simulink model "heart_model"  (Simulink 8.5)
settings: Solver=ode3  StartTime=0.0  StopTime=size(sasignal,1)  FixedStep=1  RelTol=1e-6  AbsTol=1e-6
undefined symbols (not defined in the file or in its folder): beta1, beta3, beta4, delay, gain
libraries: simulink x40, dspsrcs4 x1
(part 2 of 5)

== system heart_model/Heart Model/VENTRICLE/LV (20) ==
  stim : Inport
  I_st : Inport  Port=2
  vin : Inport  Port=3
  win : Inport  Port=4
  Data Type Conversion : DataTypeConversion  OutMin=[0]  OutMax=[1]  OutDataTypeStr=double  LockScale=on
  Data Type Conversion1 : DataTypeConversion  OutMin=[0]  OutMax=[1]  OutDataTypeStr=double  LockScale=on
  Data Type Conversion2 : DataTypeConversion  OutMin=[0]  OutMax=[1]  OutDataTypeStr=double  LockScale=on
  Event generator : Stateflow chart  TreatAsAtomicUnit=on
  Hybrid set : Stateflow chart  TreatAsAtomicUnit=on
  Mux : Mux  Inputs=5
  Subsystem3 : Subsystem
  vout : Outport
  wires:
  Data Type Conversion2/1 -> Mux/3
  Data Type Conversion1/1 -> Mux/2
  Event generator/3(event3) -> Data Type Conversion2/1
  Event generator/2(event2) -> Data Type Conversion1/1
  Data Type Conversion/1 -> Mux/1
  Event generator/1(event1) -> Data Type Conversion/1
  stim/1 -> Mux/5, Mux/4
  Mux/1 -> Hybrid set/Trigger
  win/1 -> Subsystem3/7(win)
  vin/1 -> Subsystem3/6(vin)
  Hybrid set/3(vno) -> Subsystem3/5(vno)
  I_st/1 -> Subsystem3/4(I_st)
  Subsystem3/1(v) -> vout/1
  Hybrid set/1(q) -> Subsystem3/1(q)
  Subsystem3/2(vnext) -> Event generator/1(v), Hybrid set/1(v)
  Hybrid set/2(vreset) -> Subsystem3/2(vreset)
  Hybrid set/4(reset) -> Subsystem3/3(reset)

== system heart_model/Heart Model/VENTRICLE/LVA (16) ==
  stim : Inport
  I_st : Inport  Port=2
  vin : Inport  Port=3
  win : Inport  Port=4
  Data Type Conversion : DataTypeConversion  OutMin=[0]  OutMax=[1]  OutDataTypeStr=double  LockScale=on
  Data Type Conversion1 : DataTypeConversion  OutMin=[0]  OutMax=[1]  OutDataTypeStr=double  LockScale=on
  Data Type Conversion2 : DataTypeConversion  OutMin=[0]  OutMax=[1]  OutDataTypeStr=double  LockScale=on
  Event generator : Stateflow chart  TreatAsAtomicUnit=on
  Hybrid set : Stateflow chart  TreatAsAtomicUnit=on
  Mux : Mux  Inputs=5
  Subsystem3 : Subsystem
  vout : Outport
  wires:
  Data Type Conversion2/1 -> Mux/3
  Data Type Conversion1/1 -> Mux/2
  Event generator/3(event3) -> Data Type Conversion2/1
  Event generator/2(event2) -> Data Type Conversion1/1
  Data Type Conversion/1 -> Mux/1
  Event generator/1(event1) -> Data Type Conversion/1
  stim/1 -> Mux/5, Mux/4
  Mux/1 -> Hybrid set/Trigger
  win/1 -> Subsystem3/7(win)
  vin/1 -> Subsystem3/6(vin)
  Hybrid set/3(vno) -> Subsystem3/5(vno)
  I_st/1 -> Subsystem3/4(I_st)
  Subsystem3/1(v) -> vout/1
  Hybrid set/1(q) -> Subsystem3/1(q)
  Subsystem3/2(vnext) -> Event generator/1(v), Hybrid set/1(v)
  Hybrid set/2(vreset) -> Subsystem3/2(vreset)
  Hybrid set/4(reset) -> Subsystem3/3(reset)

== system heart_model/Heart Model/VENTRICLE/LV_m (19) ==
  stim : Inport
  I_st : Inport  Port=2
  vin : Inport  Port=3
  win : Inport  Port=4
  Data Type Conversion : DataTypeConversion  OutMin=[0]  OutMax=[1]  OutDataTypeStr=double  LockScale=on
  Data Type Conversion1 : DataTypeConversion  OutMin=[0]  OutMax=[1]  OutDataTypeStr=double  LockScale=on
  Data Type Conversion2 : DataTypeConversion  OutMin=[0]  OutMax=[1]  OutDataTypeStr=double  LockScale=on
  Event generator : Stateflow chart  TreatAsAtomicUnit=on
  Hybrid set : Stateflow chart  TreatAsAtomicUnit=on
  Mux : Mux  Inputs=5
  Subsystem3 : Subsystem
  vout : Outport
  wires:
  Data Type Conversion2/1 -> Mux/3
  Data Type Conversion1/1 -> Mux/2
  Event generator/3(event3) -> Data Type Conversion2/1
  Event generator/2(event2) -> Data Type Conversion1/1
  Data Type Conversion/1 -> Mux/1
  Event generator/1(event1) -> Data Type Conversion/1
  stim/1 -> Mux/5, Mux/4
  Mux/1 -> Hybrid set/Trigger
  win/1 -> Subsystem3/7(win)
  vin/1 -> Subsystem3/6(vin)
  Hybrid set/3(vno) -> Subsystem3/5(vno)
  I_st/1 -> Subsystem3/4(I_st)
  Subsystem3/1(v) -> vout/1
  Hybrid set/1(q) -> Subsystem3/1(q)
  Subsystem3/2(vnext) -> Event generator/1(v), Hybrid set/1(v)
  Hybrid set/2(vreset) -> Subsystem3/2(vreset)
  Hybrid set/4(reset) -> Subsystem3/3(reset)

== system heart_model/Heart Model/VENTRICLE/RBB (12) ==
  stim : Inport
  I_st : Inport  Port=2
  vin : Inport  Port=3
  win : Inport  Port=4
  Data Type Conversion : DataTypeConversion  OutMin=[0]  OutMax=[1]  OutDataTypeStr=double  LockScale=on
  Data Type Conversion1 : DataTypeConversion  OutMin=[0]  OutMax=[1]  OutDataTypeStr=double  LockScale=on
  Data Type Conversion2 : DataTypeConversion  OutMin=[0]  OutMax=[1]  OutDataTypeStr=double  LockScale=on
  Event generator : Stateflow chart  TreatAsAtomicUnit=on
  Hybrid set : Stateflow chart  TreatAsAtomicUnit=on
  Mux : Mux  Inputs=5
  Subsystem3 : Subsystem
  vout : Outport
  wires:
  Data Type Conversion2/1 -> Mux/3
  Data Type Conversion1/1 -> Mux/2
  Event generator/3(event3) -> Data Type Conversion2/1
  Event generator/2(event2) -> Data Type Conversion1/1
  Data Type Conversion/1 -> Mux/1
  Event generator/1(event1) -> Data Type Conversion/1
  stim/1 -> Mux/5, Mux/4
  Mux/1 -> Hybrid set/Trigger
  win/1 -> Subsystem3/7(win)
  vin/1 -> Subsystem3/6(vin)
  Hybrid set/3(vno) -> Subsystem3/5(vno)
  I_st/1 -> Subsystem3/4(I_st)
  Subsystem3/1(v) -> vout/1
  Hybrid set/1(q) -> Subsystem3/1(q)
  Subsystem3/2(vnext) -> Event generator/1(v), Hybrid set/1(v)
  Hybrid set/2(vreset) -> Subsystem3/2(vreset)
  Hybrid set/4(reset) -> Subsystem3/3(reset)

== system heart_model/Heart Model/VENTRICLE/RBB_m (11) ==
  stim : Inport
  I_st : Inport  Port=2
  vin : Inport  Port=3
  win : Inport  Port=4
  Data Type Conversion : DataTypeConversion  OutMin=[0]  OutMax=[1]  OutDataTypeStr=double  LockScale=on
  Data Type Conversion1 : DataTypeConversion  OutMin=[0]  OutMax=[1]  OutDataTypeStr=double  LockScale=on
  Data Type Conversion2 : DataTypeConversion  OutMin=[0]  OutMax=[1]  OutDataTypeStr=double  LockScale=on
  Event generator : Stateflow chart  TreatAsAtomicUnit=on
  Hybrid set : Stateflow chart  TreatAsAtomicUnit=on
  Mux : Mux  Inputs=5
  Subsystem3 : Subsystem
  vout : Outport
  wires:
  Data Type Conversion2/1 -> Mux/3
  Data Type Conversion1/1 -> Mux/2
  Event generator/3(event3) -> Data Type Conversion2/1
  Event generator/2(event2) -> Data Type Conversion1/1
  Data Type Conversion/1 -> Mux/1
  Event generator/1(event1) -> Data Type Conversion/1
  stim/1 -> Mux/5, Mux/4
  Mux/1 -> Hybrid set/Trigger
  win/1 -> Subsystem3/7(win)
  vin/1 -> Subsystem3/6(vin)
  Hybrid set/3(vno) -> Subsystem3/5(vno)
  I_st/1 -> Subsystem3/4(I_st)
  Subsystem3/1(v) -> vout/1
  Hybrid set/1(q) -> Subsystem3/1(q)
  Subsystem3/2(vnext) -> Event generator/1(v), Hybrid set/1(v)
  Hybrid set/2(vreset) -> Subsystem3/2(vreset)
  Hybrid set/4(reset) -> Subsystem3/3(reset)

== system heart_model/Heart Model/VENTRICLE/RV (18) ==
  stim : Inport
  I_st : Inport  Port=2
  vin : Inport  Port=3
  win : Inport  Port=4
  Data Type Conversion : DataTypeConversion  OutMin=[0]  OutMax=[1]  OutDataTypeStr=double  LockScale=on
  Data Type Conversion1 : DataTypeConversion  OutMin=[0]  OutMax=[1]  OutDataTypeStr=double  LockScale=on
  Data Type Conversion2 : DataTypeConversion  OutMin=[0]  OutMax=[1]  OutDataTypeStr=double  LockScale=on
  Event generator : Stateflow chart  TreatAsAtomicUnit=on
  Hybrid set : Stateflow chart  TreatAsAtomicUnit=on
  Mux : Mux  Inputs=5
  Subsystem3 : Subsystem
  vout : Outport
  wires:
  Data Type Conversion2/1 -> Mux/3
  Data Type Conversion1/1 -> Mux/2
  Event generator/3(event3) -> Data Type Conversion2/1
  Event generator/2(event2) -> Data Type Conversion1/1
  Data Type Conversion/1 -> Mux/1
  Event generator/1(event1) -> Data Type Conversion/1
  stim/1 -> Mux/5, Mux/4
  Mux/1 -> Hybrid set/Trigger
  win/1 -> Subsystem3/7(win)
  vin/1 -> Subsystem3/6(vin)
  Hybrid set/3(vno) -> Subsystem3/5(vno)
  I_st/1 -> Subsystem3/4(I_st)
  Subsystem3/1(v) -> vout/1
  Hybrid set/1(q) -> Subsystem3/1(q)
  Subsystem3/2(vnext) -> Event generator/1(v), Hybrid set/1(v)
  Hybrid set/2(vreset) -> Subsystem3/2(vreset)
  Hybrid set/4(reset) -> Subsystem3/3(reset)

== system heart_model/Heart Model/VENTRICLE/RVA (15) ==
  stim : Inport
  I_st : Inport  Port=2
  vin : Inport  Port=3
  win : Inport  Port=4
  Data Type Conversion : DataTypeConversion  OutMin=[0]  OutMax=[1]  OutDataTypeStr=double  LockScale=on
  Data Type Conversion1 : DataTypeConversion  OutMin=[0]  OutMax=[1]  OutDataTypeStr=double  LockScale=on
  Data Type Conversion2 : DataTypeConversion  OutMin=[0]  OutMax=[1]  OutDataTypeStr=double  LockScale=on
  Event generator : Stateflow chart  TreatAsAtomicUnit=on
  Hybrid set : Stateflow chart  TreatAsAtomicUnit=on
  Mux : Mux  Inputs=5
  Subsystem3 : Subsystem
  vout : Outport
  wires:
  Data Type Conversion2/1 -> Mux/3
  Data Type Conversion1/1 -> Mux/2
  Event generator/3(event3) -> Data Type Conversion2/1
  Event generator/2(event2) -> Data Type Conversion1/1
  Data Type Conversion/1 -> Mux/1
  Event generator/1(event1) -> Data Type Conversion/1
  stim/1 -> Mux/5, Mux/4
  Mux/1 -> Hybrid set/Trigger
  win/1 -> Subsystem3/7(win)
  vin/1 -> Subsystem3/6(vin)
  Hybrid set/3(vno) -> Subsystem3/5(vno)
  I_st/1 -> Subsystem3/4(I_st)
  Subsystem3/1(v) -> vout/1
  Hybrid set/1(q) -> Subsystem3/1(q)
  Subsystem3/2(vnext) -> Event generator/1(v), Hybrid set/1(v)
  Hybrid set/2(vreset) -> Subsystem3/2(vreset)
  Hybrid set/4(reset) -> Subsystem3/3(reset)

== system heart_model/Heart Model/VENTRICLE/RV_m (17) ==
  stim : Inport
  I_st : Inport  Port=2
  vin : Inport  Port=3
  win : Inport  Port=4
  Data Type Conversion : DataTypeConversion  OutMin=[0]  OutMax=[1]  OutDataTypeStr=double  LockScale=on
  Data Type Conversion1 : DataTypeConversion  OutMin=[0]  OutMax=[1]  OutDataTypeStr=double  LockScale=on
  Data Type Conversion2 : DataTypeConversion  OutMin=[0]  OutMax=[1]  OutDataTypeStr=double  LockScale=on
  Event generator : Stateflow chart  TreatAsAtomicUnit=on
  Hybrid set : Stateflow chart  TreatAsAtomicUnit=on
  Mux : Mux  Inputs=5
  Subsystem3 : Subsystem
  vout : Outport
  wires:
  Data Type Conversion2/1 -> Mux/3
  Data Type Conversion1/1 -> Mux/2
  Event generator/3(event3) -> Data Type Conversion2/1
  Event generator/2(event2) -> Data Type Conversion1/1
  Data Type Conversion/1 -> Mux/1
  Event generator/1(event1) -> Data Type Conversion/1
  stim/1 -> Mux/5, Mux/4
  Mux/1 -> Hybrid set/Trigger
  win/1 -> Subsystem3/7(win)
  vin/1 -> Subsystem3/6(vin)
  Hybrid set/3(vno) -> Subsystem3/5(vno)
  I_st/1 -> Subsystem3/4(I_st)
  Subsystem3/1(v) -> vout/1
  Hybrid set/1(q) -> Subsystem3/1(q)
  Subsystem3/2(vnext) -> Event generator/1(v), Hybrid set/1(v)
  Hybrid set/2(vreset) -> Subsystem3/2(vreset)
  Hybrid set/4(reset) -> Subsystem3/3(reset)

== system heart_model/Heart Model/VENTRICLE/SEP_LV (27) ==
  stim : Inport
  I_st : Inport  Port=2
  vin : Inport  Port=3
  win : Inport  Port=4
  Data Type Conversion : DataTypeConversion  OutMin=[0]  OutMax=[1]  OutDataTypeStr=double  LockScale=on
  Data Type Conversion1 : DataTypeConversion  OutMin=[0]  OutMax=[1]  OutDataTypeStr=double  LockScale=on
  Data Type Conversion2 : DataTypeConversion  OutMin=[0]  OutMax=[1]  OutDataTypeStr=double  LockScale=on
  Event generator : Stateflow chart  TreatAsAtomicUnit=on
  Hybrid set : Stateflow chart  TreatAsAtomicUnit=on
  Mux : Mux  Inputs=5
  Subsystem3 : Subsystem
  vout : Outport
  wires:
  Data Type Conversion2/1 -> Mux/3
  Data Type Conversion1/1 -> Mux/2
  Event generator/3(event3) -> Data Type Conversion2/1
  Event generator/2(event2) -> Data Type Conversion1/1
  Data Type Conversion/1 -> Mux/1
  Event generator/1(event1) -> Data Type Conversion/1
  stim/1 -> Mux/5, Mux/4
  Mux/1 -> Hybrid set/Trigger
  win/1 -> Subsystem3/7(win)
  vin/1 -> Subsystem3/6(vin)
  Hybrid set/3(vno) -> Subsystem3/5(vno)
  I_st/1 -> Subsystem3/4(I_st)
  Subsystem3/1(v) -> vout/1
  Hybrid set/1(q) -> Subsystem3/1(q)
  Subsystem3/2(vnext) -> Event generator/1(v), Hybrid set/1(v)
  Hybrid set/2(vreset) -> Subsystem3/2(vreset)
  Hybrid set/4(reset) -> Subsystem3/3(reset)

== system heart_model/Heart Model/VENTRICLE/SEP_LV_m (26) ==
  stim : Inport
  I_st : Inport  Port=2
  vin : Inport  Port=3
  win : Inport  Port=4
  Data Type Conversion : DataTypeConversion  OutMin=[0]  OutMax=[1]  OutDataTypeStr=double  LockScale=on
  Data Type Conversion1 : DataTypeConversion  OutMin=[0]  OutMax=[1]  OutDataTypeStr=double  LockScale=on
  Data Type Conversion2 : DataTypeConversion  OutMin=[0]  OutMax=[1]  OutDataTypeStr=double  LockScale=on
  Event generator : Stateflow chart  TreatAsAtomicUnit=on
  Hybrid set : Stateflow chart  TreatAsAtomicUnit=on
  Mux : Mux  Inputs=5
  Subsystem3 : Subsystem
  vout : Outport
  wires:
  Data Type Conversion2/1 -> Mux/3
  Data Type Conversion1/1 -> Mux/2
  Event generator/3(event3) -> Data Type Conversion2/1
  Event generator/2(event2) -> Data Type Conversion1/1
  Data Type Conversion/1 -> Mux/1
  Event generator/1(event1) -> Data Type Conversion/1
  stim/1 -> Mux/5, Mux/4
  Mux/1 -> Hybrid set/Trigger
  win/1 -> Subsystem3/7(win)
  vin/1 -> Subsystem3/6(vin)
  Hybrid set/3(vno) -> Subsystem3/5(vno)
  I_st/1 -> Subsystem3/4(I_st)
  Subsystem3/1(v) -> vout/1
  Hybrid set/1(q) -> Subsystem3/1(q)
  Subsystem3/2(vnext) -> Event generator/1(v), Hybrid set/1(v)
  Hybrid set/2(vreset) -> Subsystem3/2(vreset)
  Hybrid set/4(reset) -> Subsystem3/3(reset)

== system heart_model/Heart Model/VENTRICLE/SEP_RV (25) ==
  stim : Inport
  I_st : Inport  Port=2
  vin : Inport  Port=3
  win : Inport  Port=4
  Data Type Conversion : DataTypeConversion  OutMin=[0]  OutMax=[1]  OutDataTypeStr=double  LockScale=on
  Data Type Conversion1 : DataTypeConversion  OutMin=[0]  OutMax=[1]  OutDataTypeStr=double  LockScale=on
  Data Type Conversion2 : DataTypeConversion  OutMin=[0]  OutMax=[1]  OutDataTypeStr=double  LockScale=on
  Event generator : Stateflow chart  TreatAsAtomicUnit=on
  Hybrid set : Stateflow chart  TreatAsAtomicUnit=on
  Mux : Mux  Inputs=5
  Subsystem3 : Subsystem
  vout : Outport
  wires:
  Data Type Conversion2/1 -> Mux/3
  Data Type Conversion1/1 -> Mux/2
  Event generator/3(event3) -> Data Type Conversion2/1
  Event generator/2(event2) -> Data Type Conversion1/1
  Data Type Conversion/1 -> Mux/1
  Event generator/1(event1) -> Data Type Conversion/1
  stim/1 -> Mux/5, Mux/4
  Mux/1 -> Hybrid set/Trigger
  win/1 -> Subsystem3/7(win)
  vin/1 -> Subsystem3/6(vin)
  Hybrid set/3(vno) -> Subsystem3/5(vno)
  I_st/1 -> Subsystem3/4(I_st)
  Subsystem3/1(v) -> vout/1
  Hybrid set/1(q) -> Subsystem3/1(q)
  Subsystem3/2(vnext) -> Event generator/1(v), Hybrid set/1(v)
  Hybrid set/2(vreset) -> Subsystem3/2(vreset)
  Hybrid set/4(reset) -> Subsystem3/3(reset)

== system heart_model/Heart Model/VENTRICLE/SEP_RV_m (24) ==
  stim : Inport
  I_st : Inport  Port=2
  vin : Inport  Port=3
  win : Inport  Port=4
  Data Type Conversion : DataTypeConversion  OutMin=[0]  OutMax=[1]  OutDataTypeStr=double  LockScale=on
  Data Type Conversion1 : DataTypeConversion  OutMin=[0]  OutMax=[1]  OutDataTypeStr=double  LockScale=on
  Data Type Conversion2 : DataTypeConversion  OutMin=[0]  OutMax=[1]  OutDataTypeStr=double  LockScale=on
  Event generator : Stateflow chart  TreatAsAtomicUnit=on
  Hybrid set : Stateflow chart  TreatAsAtomicUnit=on
  Mux : Mux  Inputs=5
  Subsystem3 : Subsystem
  vout : Outport
  wires:
  Data Type Conversion2/1 -> Mux/3
  Data Type Conversion1/1 -> Mux/2
  Event generator/3(event3) -> Data Type Conversion2/1
  Event generator/2(event2) -> Data Type Conversion1/1
  Data Type Conversion/1 -> Mux/1
  Event generator/1(event1) -> Data Type Conversion/1
  stim/1 -> Mux/5, Mux/4
  Mux/1 -> Hybrid set/Trigger
  win/1 -> Subsystem3/7(win)
  vin/1 -> Subsystem3/6(vin)
  Hybrid set/3(vno) -> Subsystem3/5(vno)
  I_st/1 -> Subsystem3/4(I_st)
  Subsystem3/1(v) -> vout/1
  Hybrid set/1(q) -> Subsystem3/1(q)
  Subsystem3/2(vnext) -> Event generator/1(v), Hybrid set/1(v)
  Hybrid set/2(vreset) -> Subsystem3/2(vreset)
  Hybrid set/4(reset) -> Subsystem3/3(reset)

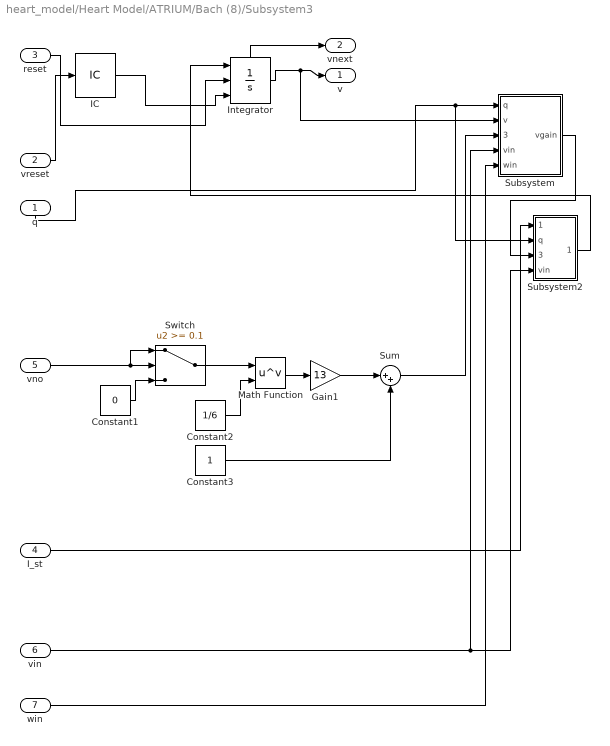
== system heart_model/Heart Model/ATRIUM/Bach (8)/Subsystem3 ==
  q : Inport
  vreset : Inport  Port=2
  reset : Inport  Port=3
  I_st : Inport  Port=4
  vno : Inport  Port=5
  vin : Inport  Port=6
  win : Inport  Port=7
  Constant1 : Constant  Value=0
  Constant2 : Constant  Value=1/6
  Constant3 : Constant
  Gain1 : Gain  Gain=13
  IC : InitialCondition  Value=0
  Integrator : Integrator  ExternalReset=either  InitialConditionSource=external  LimitOutput=on  UpperSaturationLimit=138  ShowStatePort=on
  Math Function : Math  Operator=pow  SaturateOnIntegerOverflow=on
  Subsystem : Subsystem
  Subsystem2 : Subsystem
  Sum : Sum  Inputs=|++
  Switch : Switch  Threshold=0.1
  v : Outport
  vnext : Outport  Port=2
  wires:
  win/1 -> Subsystem/5(win)
  vin/1 -> Subsystem/4(vin), Subsystem2/4(vin)
  Integrator/State -> vnext/1
  Constant1/1 -> Switch/3
  vno/1 -> Switch/1, Switch/2
  Sum/1 -> Subsystem/3(f(vno))
  Switch/1 -> Math Function/1
  Constant3/1 -> Sum/2
  Gain1/1 -> Sum/1
  Math Function/1 -> Gain1/1
  Constant2/1 -> Math Function/2
  I_st/1 -> Subsystem2/1(I_st)
  reset/1 -> Integrator/2
  vreset/1 -> IC/1
  Subsystem2/1(vint) -> Integrator/1
  Subsystem/1(vgain) -> Subsystem2/3(vgain)
  Integrator/1 -> Subsystem/2(v), v/1
  IC/1 -> Integrator/3
  q/1 -> Subsystem/1(q), Subsystem2/2(q)

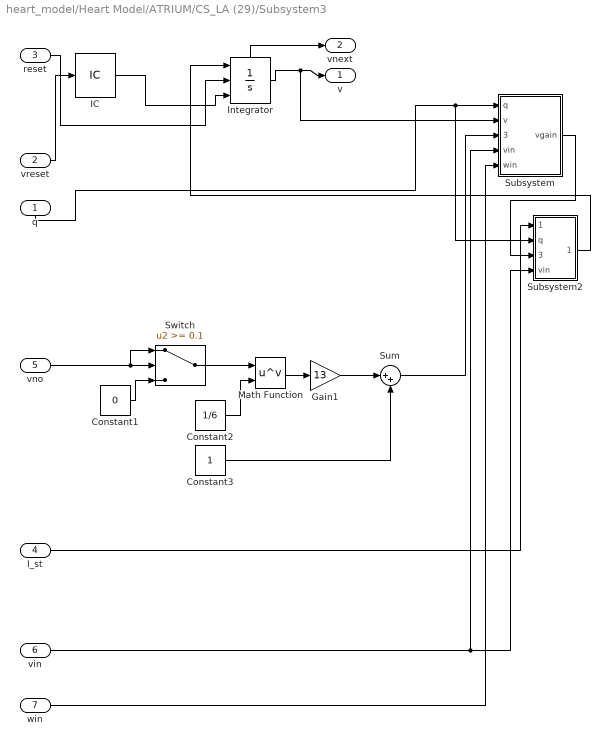
== system heart_model/Heart Model/ATRIUM/CS_LA (29)/Subsystem3 ==
  q : Inport
  vreset : Inport  Port=2
  reset : Inport  Port=3
  I_st : Inport  Port=4
  vno : Inport  Port=5
  vin : Inport  Port=6
  win : Inport  Port=7
  Constant1 : Constant  Value=0
  Constant2 : Constant  Value=1/6
  Constant3 : Constant
  Gain1 : Gain  Gain=13
  IC : InitialCondition  Value=0
  Integrator : Integrator  ExternalReset=either  InitialConditionSource=external  LimitOutput=on  UpperSaturationLimit=138  ShowStatePort=on
  Math Function : Math  Operator=pow  SaturateOnIntegerOverflow=on
  Subsystem : Subsystem
  Subsystem2 : Subsystem
  Sum : Sum  Inputs=|++
  Switch : Switch  Threshold=0.1
  v : Outport
  vnext : Outport  Port=2
  wires:
  win/1 -> Subsystem/5(win)
  vin/1 -> Subsystem/4(vin), Subsystem2/4(vin)
  Integrator/State -> vnext/1
  Constant1/1 -> Switch/3
  vno/1 -> Switch/1, Switch/2
  Sum/1 -> Subsystem/3(f(vno))
  Switch/1 -> Math Function/1
  Constant3/1 -> Sum/2
  Gain1/1 -> Sum/1
  Math Function/1 -> Gain1/1
  Constant2/1 -> Math Function/2
  I_st/1 -> Subsystem2/1(I_st)
  reset/1 -> Integrator/2
  vreset/1 -> IC/1
  Subsystem2/1(vint) -> Integrator/1
  Subsystem/1(vgain) -> Subsystem2/3(vgain)
  Integrator/1 -> Subsystem/2(v), v/1
  IC/1 -> Integrator/3
  q/1 -> Subsystem/1(q), Subsystem2/2(q)

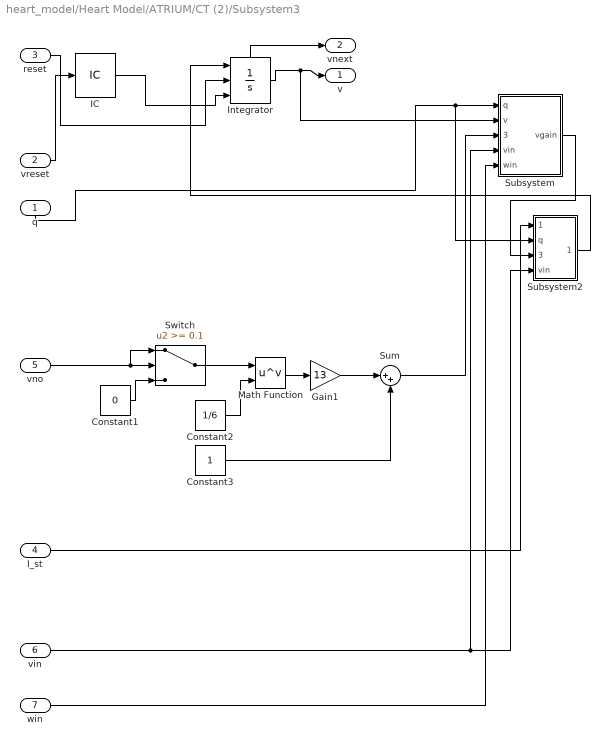
== system heart_model/Heart Model/ATRIUM/CT (2)/Subsystem3 ==
  q : Inport
  vreset : Inport  Port=2
  reset : Inport  Port=3
  I_st : Inport  Port=4
  vno : Inport  Port=5
  vin : Inport  Port=6
  win : Inport  Port=7
  Constant1 : Constant  Value=0
  Constant2 : Constant  Value=1/6
  Constant3 : Constant
  Gain1 : Gain  Gain=13
  IC : InitialCondition  Value=0
  Integrator : Integrator  ExternalReset=either  InitialConditionSource=external  LimitOutput=on  UpperSaturationLimit=138  ShowStatePort=on
  Math Function : Math  Operator=pow  SaturateOnIntegerOverflow=on
  Subsystem : Subsystem
  Subsystem2 : Subsystem
  Sum : Sum  Inputs=|++
  Switch : Switch  Threshold=0.1
  v : Outport
  vnext : Outport  Port=2
  wires:
  win/1 -> Subsystem/5(win)
  vin/1 -> Subsystem/4(vin), Subsystem2/4(vin)
  Integrator/State -> vnext/1
  Constant1/1 -> Switch/3
  vno/1 -> Switch/1, Switch/2
  Sum/1 -> Subsystem/3(f(vno))
  Switch/1 -> Math Function/1
  Constant3/1 -> Sum/2
  Gain1/1 -> Sum/1
  Math Function/1 -> Gain1/1
  Constant2/1 -> Math Function/2
  I_st/1 -> Subsystem2/1(I_st)
  reset/1 -> Integrator/2
  vreset/1 -> IC/1
  Subsystem2/1(vint) -> Integrator/1
  Subsystem/1(vgain) -> Subsystem2/3(vgain)
  Integrator/1 -> Subsystem/2(v), v/1
  IC/1 -> Integrator/3
  q/1 -> Subsystem/1(q), Subsystem2/2(q)

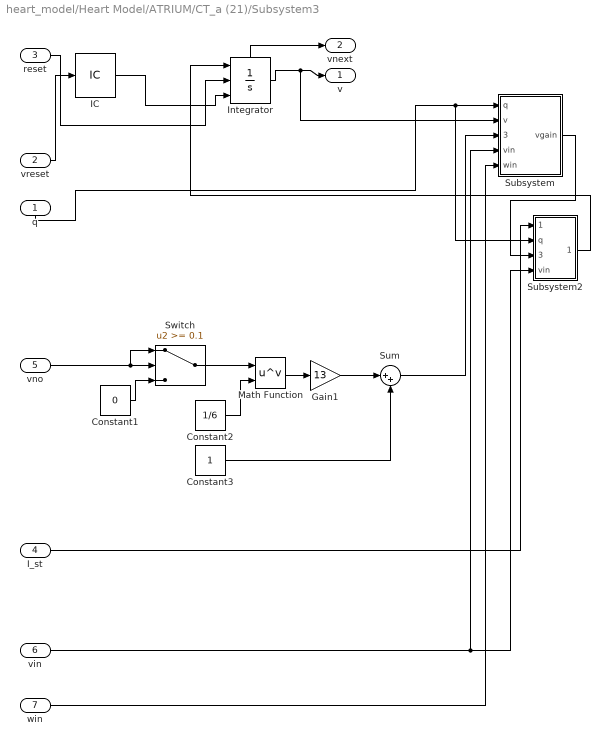
== system heart_model/Heart Model/ATRIUM/CT_a (21)/Subsystem3 ==
  q : Inport
  vreset : Inport  Port=2
  reset : Inport  Port=3
  I_st : Inport  Port=4
  vno : Inport  Port=5
  vin : Inport  Port=6
  win : Inport  Port=7
  Constant1 : Constant  Value=0
  Constant2 : Constant  Value=1/6
  Constant3 : Constant
  Gain1 : Gain  Gain=13
  IC : InitialCondition  Value=0
  Integrator : Integrator  ExternalReset=either  InitialConditionSource=external  LimitOutput=on  UpperSaturationLimit=138  ShowStatePort=on
  Math Function : Math  Operator=pow  SaturateOnIntegerOverflow=on
  Subsystem : Subsystem
  Subsystem2 : Subsystem
  Sum : Sum  Inputs=|++
  Switch : Switch  Threshold=0.1
  v : Outport
  vnext : Outport  Port=2
  wires:
  win/1 -> Subsystem/5(win)
  vin/1 -> Subsystem/4(vin), Subsystem2/4(vin)
  Integrator/State -> vnext/1
  Constant1/1 -> Switch/3
  vno/1 -> Switch/1, Switch/2
  Sum/1 -> Subsystem/3(f(vno))
  Switch/1 -> Math Function/1
  Constant3/1 -> Sum/2
  Gain1/1 -> Sum/1
  Math Function/1 -> Gain1/1
  Constant2/1 -> Math Function/2
  I_st/1 -> Subsystem2/1(I_st)
  reset/1 -> Integrator/2
  vreset/1 -> IC/1
  Subsystem2/1(vint) -> Integrator/1
  Subsystem/1(vgain) -> Subsystem2/3(vgain)
  Integrator/1 -> Subsystem/2(v), v/1
  IC/1 -> Integrator/3
  q/1 -> Subsystem/1(q), Subsystem2/2(q)

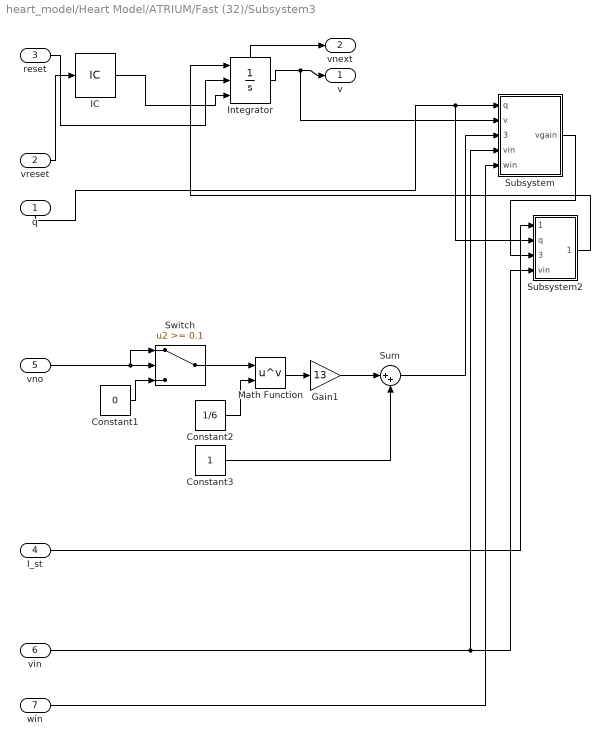
== system heart_model/Heart Model/ATRIUM/Fast (32)/Subsystem3 ==
  q : Inport
  vreset : Inport  Port=2
  reset : Inport  Port=3
  I_st : Inport  Port=4
  vno : Inport  Port=5
  vin : Inport  Port=6
  win : Inport  Port=7
  Constant1 : Constant  Value=0
  Constant2 : Constant  Value=1/6
  Constant3 : Constant
  Gain1 : Gain  Gain=13
  IC : InitialCondition  Value=0
  Integrator : Integrator  ExternalReset=either  InitialConditionSource=external  LimitOutput=on  UpperSaturationLimit=138  ShowStatePort=on
  Math Function : Math  Operator=pow  SaturateOnIntegerOverflow=on
  Subsystem : Subsystem
  Subsystem2 : Subsystem
  Sum : Sum  Inputs=|++
  Switch : Switch  Threshold=0.1
  v : Outport
  vnext : Outport  Port=2
  wires:
  win/1 -> Subsystem/5(win)
  vin/1 -> Subsystem/4(vin), Subsystem2/4(vin)
  Integrator/State -> vnext/1
  Constant1/1 -> Switch/3
  vno/1 -> Switch/1, Switch/2
  Sum/1 -> Subsystem/3(f(vno))
  Switch/1 -> Math Function/1
  Constant3/1 -> Sum/2
  Gain1/1 -> Sum/1
  Math Function/1 -> Gain1/1
  Constant2/1 -> Math Function/2
  I_st/1 -> Subsystem2/1(I_st)
  reset/1 -> Integrator/2
  vreset/1 -> IC/1
  Subsystem2/1(vint) -> Integrator/1
  Subsystem/1(vgain) -> Subsystem2/3(vgain)
  Integrator/1 -> Subsystem/2(v), v/1
  IC/1 -> Integrator/3
  q/1 -> Subsystem/1(q), Subsystem2/2(q)

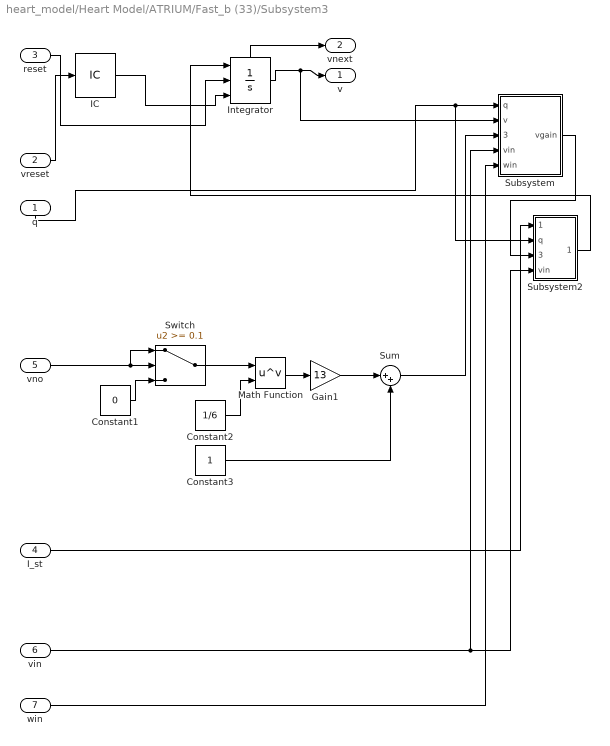
== system heart_model/Heart Model/ATRIUM/Fast_b (33)/Subsystem3 ==
  q : Inport
  vreset : Inport  Port=2
  reset : Inport  Port=3
  I_st : Inport  Port=4
  vno : Inport  Port=5
  vin : Inport  Port=6
  win : Inport  Port=7
  Constant1 : Constant  Value=0
  Constant2 : Constant  Value=1/6
  Constant3 : Constant
  Gain1 : Gain  Gain=13
  IC : InitialCondition  Value=0
  Integrator : Integrator  ExternalReset=either  InitialConditionSource=external  LimitOutput=on  UpperSaturationLimit=138  ShowStatePort=on
  Math Function : Math  Operator=pow  SaturateOnIntegerOverflow=on
  Subsystem : Subsystem
  Subsystem2 : Subsystem
  Sum : Sum  Inputs=|++
  Switch : Switch  Threshold=0.1
  v : Outport
  vnext : Outport  Port=2
  wires:
  win/1 -> Subsystem/5(win)
  vin/1 -> Subsystem/4(vin), Subsystem2/4(vin)
  Integrator/State -> vnext/1
  Constant1/1 -> Switch/3
  vno/1 -> Switch/1, Switch/2
  Sum/1 -> Subsystem/3(f(vno))
  Switch/1 -> Math Function/1
  Constant3/1 -> Sum/2
  Gain1/1 -> Sum/1
  Math Function/1 -> Gain1/1
  Constant2/1 -> Math Function/2
  I_st/1 -> Subsystem2/1(I_st)
  reset/1 -> Integrator/2
  vreset/1 -> IC/1
  Subsystem2/1(vint) -> Integrator/1
  Subsystem/1(vgain) -> Subsystem2/3(vgain)
  Integrator/1 -> Subsystem/2(v), v/1
  IC/1 -> Integrator/3
  q/1 -> Subsystem/1(q), Subsystem2/2(q)

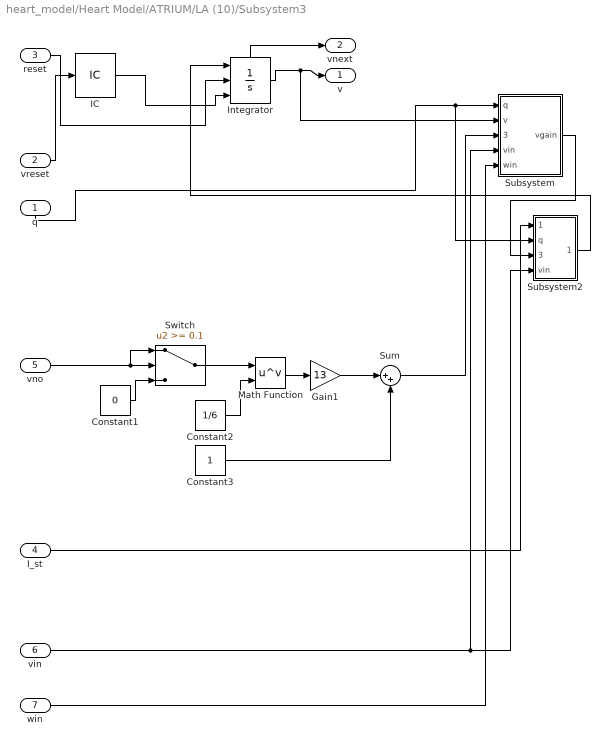
== system heart_model/Heart Model/ATRIUM/LA (10)/Subsystem3 ==
  q : Inport
  vreset : Inport  Port=2
  reset : Inport  Port=3
  I_st : Inport  Port=4
  vno : Inport  Port=5
  vin : Inport  Port=6
  win : Inport  Port=7
  Constant1 : Constant  Value=0
  Constant2 : Constant  Value=1/6
  Constant3 : Constant
  Gain1 : Gain  Gain=13
  IC : InitialCondition  Value=0
  Integrator : Integrator  ExternalReset=either  InitialConditionSource=external  LimitOutput=on  UpperSaturationLimit=138  ShowStatePort=on
  Math Function : Math  Operator=pow  SaturateOnIntegerOverflow=on
  Subsystem : Subsystem
  Subsystem2 : Subsystem
  Sum : Sum  Inputs=|++
  Switch : Switch  Threshold=0.1
  v : Outport
  vnext : Outport  Port=2
  wires:
  win/1 -> Subsystem/5(win)
  vin/1 -> Subsystem/4(vin), Subsystem2/4(vin)
  Integrator/State -> vnext/1
  Constant1/1 -> Switch/3
  vno/1 -> Switch/1, Switch/2
  Sum/1 -> Subsystem/3(f(vno))
  Switch/1 -> Math Function/1
  Constant3/1 -> Sum/2
  Gain1/1 -> Sum/1
  Math Function/1 -> Gain1/1
  Constant2/1 -> Math Function/2
  I_st/1 -> Subsystem2/1(I_st)
  reset/1 -> Integrator/2
  vreset/1 -> IC/1
  Subsystem2/1(vint) -> Integrator/1
  Subsystem/1(vgain) -> Subsystem2/3(vgain)
  Integrator/1 -> Subsystem/2(v), v/1
  IC/1 -> Integrator/3
  q/1 -> Subsystem/1(q), Subsystem2/2(q)

== system heart_model/Heart Model/ATRIUM/LA_a (9)/Subsystem3 ==
  q : Inport
  vreset : Inport  Port=2
  reset : Inport  Port=3
  I_st : Inport  Port=4
  vno : Inport  Port=5
  vin : Inport  Port=6
  win : Inport  Port=7
  Constant1 : Constant  Value=0
  Constant2 : Constant  Value=1/6
  Constant3 : Constant
  Gain1 : Gain  Gain=13
  IC : InitialCondition  Value=0
  Integrator : Integrator  ExternalReset=either  InitialConditionSource=external  LimitOutput=on  UpperSaturationLimit=138  ShowStatePort=on
  Math Function : Math  Operator=pow  SaturateOnIntegerOverflow=on
  Subsystem : Subsystem
  Subsystem2 : Subsystem
  Sum : Sum  Inputs=|++
  Switch : Switch  Threshold=0.1
  v : Outport
  vnext : Outport  Port=2
  wires:
  win/1 -> Subsystem/5(win)
  vin/1 -> Subsystem/4(vin), Subsystem2/4(vin)
  Integrator/State -> vnext/1
  Constant1/1 -> Switch/3
  vno/1 -> Switch/1, Switch/2
  Sum/1 -> Subsystem/3(f(vno))
  Switch/1 -> Math Function/1
  Constant3/1 -> Sum/2
  Gain1/1 -> Sum/1
  Math Function/1 -> Gain1/1
  Constant2/1 -> Math Function/2
  I_st/1 -> Subsystem2/1(I_st)
  reset/1 -> Integrator/2
  vreset/1 -> IC/1
  Subsystem2/1(vint) -> Integrator/1
  Subsystem/1(vgain) -> Subsystem2/3(vgain)
  Integrator/1 -> Subsystem/2(v), v/1
  IC/1 -> Integrator/3
  q/1 -> Subsystem/1(q), Subsystem2/2(q)

== system heart_model/Heart Model/ATRIUM/OS (4)/Subsystem3 ==
  q : Inport
  vreset : Inport  Port=2
  reset : Inport  Port=3
  I_st : Inport  Port=4
  vno : Inport  Port=5
  vin : Inport  Port=6
  win : Inport  Port=7
  Constant1 : Constant  Value=0
  Constant2 : Constant  Value=1/6
  Constant3 : Constant
  Gain1 : Gain  Gain=13
  IC : InitialCondition  Value=0
  Integrator : Integrator  ExternalReset=either  InitialConditionSource=external  LimitOutput=on  UpperSaturationLimit=138  ShowStatePort=on
  Math Function : Math  Operator=pow  SaturateOnIntegerOverflow=on
  Subsystem : Subsystem
  Subsystem2 : Subsystem
  Sum : Sum  Inputs=|++
  Switch : Switch  Threshold=0.1
  v : Outport
  vnext : Outport  Port=2
  wires:
  win/1 -> Subsystem/5(win)
  vin/1 -> Subsystem/4(vin)
  Integrator/State -> vnext/1
  Constant1/1 -> Switch/3
  vno/1 -> Switch/1, Switch/2
  Sum/1 -> Subsystem/3(f(vno))
  Switch/1 -> Math Function/1
  Constant3/1 -> Sum/2
  Gain1/1 -> Sum/1
  Math Function/1 -> Gain1/1
  Constant2/1 -> Math Function/2
  I_st/1 -> Subsystem2/1(I_st)
  reset/1 -> Integrator/2
  vreset/1 -> IC/1
  Subsystem2/1(vint) -> Integrator/1
  Subsystem/1(vgain) -> Subsystem2/3(vgain)
  Integrator/1 -> Subsystem/2(v), v/1
  IC/1 -> Integrator/3
  q/1 -> Subsystem/1(q), Subsystem2/2(q)

== system heart_model/Heart Model/ATRIUM/RA (23)/Subsystem3 ==
  q : Inport
  vreset : Inport  Port=2
  reset : Inport  Port=3
  I_st : Inport  Port=4
  vno : Inport  Port=5
  vin : Inport  Port=6
  win : Inport  Port=7
  Constant1 : Constant  Value=0
  Constant2 : Constant  Value=1/6
  Constant3 : Constant
  Gain1 : Gain  Gain=13
  IC : InitialCondition  Value=0
  Integrator : Integrator  ExternalReset=either  InitialConditionSource=external  LimitOutput=on  UpperSaturationLimit=138  ShowStatePort=on
  Math Function : Math  Operator=pow  SaturateOnIntegerOverflow=on
  Subsystem : Subsystem
  Subsystem2 : Subsystem
  Sum : Sum  Inputs=|++
  Switch : Switch  Threshold=0.1
  v : Outport
  vnext : Outport  Port=2
  wires:
  win/1 -> Subsystem/5(win)
  vin/1 -> Subsystem/4(vin), Subsystem2/4(vin)
  Integrator/State -> vnext/1
  Constant1/1 -> Switch/3
  vno/1 -> Switch/1, Switch/2
  Sum/1 -> Subsystem/3(f(vno))
  Switch/1 -> Math Function/1
  Constant3/1 -> Sum/2
  Gain1/1 -> Sum/1
  Math Function/1 -> Gain1/1
  Constant2/1 -> Math Function/2
  I_st/1 -> Subsystem2/1(I_st)
  reset/1 -> Integrator/2
  vreset/1 -> IC/1
  Subsystem2/1(vint) -> Integrator/1
  Subsystem/1(vgain) -> Subsystem2/3(vgain)
  Integrator/1 -> Subsystem/2(v), v/1
  IC/1 -> Integrator/3
  q/1 -> Subsystem/1(q), Subsystem2/2(q)

== system heart_model/Heart Model/ATRIUM/RA_a (22)/Subsystem3 ==
  q : Inport
  vreset : Inport  Port=2
  reset : Inport  Port=3
  I_st : Inport  Port=4
  vno : Inport  Port=5
  vin : Inport  Port=6
  win : Inport  Port=7
  Constant1 : Constant  Value=0
  Constant2 : Constant  Value=1/6
  Constant3 : Constant
  Gain1 : Gain  Gain=13
  IC : InitialCondition  Value=0
  Integrator : Integrator  ExternalReset=either  InitialConditionSource=external  LimitOutput=on  UpperSaturationLimit=138  ShowStatePort=on
  Math Function : Math  Operator=pow  SaturateOnIntegerOverflow=on
  Subsystem : Subsystem
  Subsystem2 : Subsystem
  Sum : Sum  Inputs=|++
  Switch : Switch  Threshold=0.1
  v : Outport
  vnext : Outport  Port=2
  wires:
  win/1 -> Subsystem/5(win)
  vin/1 -> Subsystem/4(vin), Subsystem2/4(vin)
  Integrator/State -> vnext/1
  Constant1/1 -> Switch/3
  vno/1 -> Switch/1, Switch/2
  Sum/1 -> Subsystem/3(f(vno))
  Switch/1 -> Math Function/1
  Constant3/1 -> Sum/2
  Gain1/1 -> Sum/1
  Math Function/1 -> Gain1/1
  Constant2/1 -> Math Function/2
  I_st/1 -> Subsystem2/1(I_st)
  reset/1 -> Integrator/2
  vreset/1 -> IC/1
  Subsystem2/1(vint) -> Integrator/1
  Subsystem/1(vgain) -> Subsystem2/3(vgain)
  Integrator/1 -> Subsystem/2(v), v/1
  IC/1 -> Integrator/3
  q/1 -> Subsystem/1(q), Subsystem2/2(q)

== system heart_model/Heart Model/ATRIUM/Slow_a (31)/Subsystem3 ==
  q : Inport
  vreset : Inport  Port=2
  reset : Inport  Port=3
  I_st : Inport  Port=4
  vno : Inport  Port=5
  vin : Inport  Port=6
  win : Inport  Port=7
  Constant1 : Constant  Value=0
  Constant2 : Constant  Value=1/6
  Constant3 : Constant
  Gain1 : Gain  Gain=13
  IC : InitialCondition  Value=0
  Integrator : Integrator  ExternalReset=either  InitialConditionSource=external  LimitOutput=on  UpperSaturationLimit=138  ShowStatePort=on
  Math Function : Math  Operator=pow  SaturateOnIntegerOverflow=on
  Subsystem : Subsystem
  Subsystem2 : Subsystem
  Sum : Sum  Inputs=|++
  Switch : Switch  Threshold=0.1
  v : Outport
  vnext : Outport  Port=2
  wires:
  win/1 -> Subsystem/5(win)
  vin/1 -> Subsystem/4(vin), Subsystem2/4(vin)
  Integrator/State -> vnext/1
  Constant1/1 -> Switch/3
  vno/1 -> Switch/1, Switch/2
  Sum/1 -> Subsystem/3(f(vno))
  Switch/1 -> Math Function/1
  Constant3/1 -> Sum/2
  Gain1/1 -> Sum/1
  Math Function/1 -> Gain1/1
  Constant2/1 -> Math Function/2
  I_st/1 -> Subsystem2/1(I_st)
  reset/1 -> Integrator/2
  vreset/1 -> IC/1
  Subsystem2/1(vint) -> Integrator/1
  Subsystem/1(vgain) -> Subsystem2/3(vgain)
  Integrator/1 -> Subsystem/2(v), v/1
  IC/1 -> Integrator/3
  q/1 -> Subsystem/1(q), Subsystem2/2(q)

== system heart_model/Heart Model/ATRIUM/Slow_b (30)/Subsystem3 ==
  q : Inport
  vreset : Inport  Port=2
  reset : Inport  Port=3
  I_st : Inport  Port=4
  vno : Inport  Port=5
  vin : Inport  Port=6
  win : Inport  Port=7
  Constant1 : Constant  Value=0
  Constant2 : Constant  Value=1/6
  Constant3 : Constant
  Gain1 : Gain  Gain=13
  IC : InitialCondition  Value=0
  Integrator : Integrator  ExternalReset=either  InitialConditionSource=external  LimitOutput=on  UpperSaturationLimit=138  ShowStatePort=on
  Math Function : Math  Operator=pow  SaturateOnIntegerOverflow=on
  Subsystem : Subsystem
  Subsystem2 : Subsystem
  Sum : Sum  Inputs=|++
  Switch : Switch  Threshold=0.1
  v : Outport
  vnext : Outport  Port=2
  wires:
  win/1 -> Subsystem/5(win)
  vin/1 -> Subsystem/4(vin), Subsystem2/4(vin)
  Integrator/State -> vnext/1
  Constant1/1 -> Switch/3
  vno/1 -> Switch/1, Switch/2
  Sum/1 -> Subsystem/3(f(vno))
  Switch/1 -> Math Function/1
  Constant3/1 -> Sum/2
  Gain1/1 -> Sum/1
  Math Function/1 -> Gain1/1
  Constant2/1 -> Math Function/2
  I_st/1 -> Subsystem2/1(I_st)
  reset/1 -> Integrator/2
  vreset/1 -> IC/1
  Subsystem2/1(vint) -> Integrator/1
  Subsystem/1(vgain) -> Subsystem2/3(vgain)
  Integrator/1 -> Subsystem/2(v), v/1
  IC/1 -> Integrator/3
  q/1 -> Subsystem/1(q), Subsystem2/2(q)

== system heart_model/Heart Model/AV (3)/Subsystem3/Subsystem ==
  q : Inport
  v : Inport  Port=2
  f(vno) : Inport  Port=3
  vin : Inport  Port=4
  win : Inport  Port=5
  Gain3 : Gain  Gain=-1
  Multiport Switch : MultiPortSwitch  Inputs=4
  Product : Product  RndMeth=Zero
  Product1 : Product  RndMeth=Zero
  Sum : Sum  Inputs=|++
  Sum1 : Sum  Inputs=|++
  beta1 : Gain  Gain=beta1(3)
  beta3 : Gain  Gain=beta3(3)
  beta4 : Gain  Gain=beta4(3)
  vgain : Outport
  wires:
  Gain3/1 -> Product1/2
  Product1/1 -> Multiport Switch/3, Sum1/2
  Sum1/1 -> Multiport Switch/2
  Sum/1 -> Sum1/1
  win/1 -> Gain3/1
  vin/1 -> Sum/1
  beta1/1 -> Sum/2
  f(vno)/1 -> Product/2
  beta4/1 -> Product/1
  Product/1 -> Multiport Switch/5
  v/1 -> Product1/1, beta4/1, beta3/1, beta1/1
  beta3/1 -> Multiport Switch/4
  Multiport Switch/1 -> vgain/1
  q/1 -> Multiport Switch/1

== system heart_model/Heart Model/AV (3)/Subsystem3/Subsystem2 ==
  I_st : Inport
  q : Inport  Port=2
  vgain : Inport  Port=3
  vin : Inport  Port=4
  Compare To Constant : simulink/Logic and Bit Operations/Compare To Constant  relop===  const=2  OutDataTypeStr=uint8
  Sum : Sum  Inputs=|++
  Sum1 : Sum  Inputs=|++
  Switch : Switch  Criteria=u2 ~= 0
  vint : Outport
  wires:
  Sum1/1 -> Switch/1
  Sum/1 -> Sum1/2
  vin/1 -> Sum/2
  I_st/1 -> Sum/1
  vgain/1 -> Sum1/1, Switch/3
  Switch/1 -> vint/1
  q/1 -> Compare To Constant/1
  Compare To Constant/1 -> Switch/2

== system heart_model/Heart Model/SA (1)/Subsystem3/Subsystem ==
  q : Inport
  v : Inport  Port=2
  f(vno) : Inport  Port=3
  vin : Inport  Port=4
  win : Inport  Port=5
  Gain3 : Gain  Gain=-1
  Multiport Switch : MultiPortSwitch  Inputs=4
  Product : Product  RndMeth=Zero
  Product1 : Product  RndMeth=Zero
  Sum : Sum  Inputs=|++
  Sum1 : Sum  Inputs=|++
  beta1 : Gain  Gain=beta1(1)
  beta3 : Gain  Gain=beta3(1)
  beta4 : Gain  Gain=beta4(1)
  vgain : Outport
  wires:
  Gain3/1 -> Product1/2
  Product1/1 -> Multiport Switch/3, Sum1/2
  Sum1/1 -> Multiport Switch/2
  Sum/1 -> Sum1/1
  win/1 -> Gain3/1
  vin/1 -> Sum/1
  beta1/1 -> Sum/2
  f(vno)/1 -> Product/2
  beta4/1 -> Product/1
  Product/1 -> Multiport Switch/5
  v/1 -> Product1/1, beta4/1, beta3/1, beta1/1
  beta3/1 -> Multiport Switch/4
  Multiport Switch/1 -> vgain/1
  q/1 -> Multiport Switch/1

== system heart_model/Heart Model/SA (1)/Subsystem3/Subsystem2 ==
  I_st : Inport
  q : Inport  Port=2
  vgain : Inport  Port=3
  vin : Inport  Port=4
  Compare To Constant : simulink/Logic and Bit Operations/Compare To Constant  relop===  const=2  OutDataTypeStr=uint8
  Sum : Sum  Inputs=|++
  Sum1 : Sum  Inputs=|++
  Switch : Switch  Criteria=u2 ~= 0
  vint : Outport
  wires:
  Sum1/1 -> Switch/1
  Sum/1 -> Sum1/2
  vin/1 -> Sum/2
  I_st/1 -> Sum/1
  vgain/1 -> Sum1/1, Switch/3
  Switch/1 -> vint/1
  q/1 -> Compare To Constant/1
  Compare To Constant/1 -> Switch/2

== system heart_model/Heart Model/VENTRICLE/CS_LV (28)/Subsystem3 ==
  q : Inport
  vreset : Inport  Port=2
  reset : Inport  Port=3
  I_st : Inport  Port=4
  vno : Inport  Port=5
  vin : Inport  Port=6
  win : Inport  Port=7
  Constant1 : Constant  Value=0
  Constant2 : Constant  Value=1/6
  Constant3 : Constant
  Gain1 : Gain  Gain=13
  IC : InitialCondition  Value=0
  Integrator : Integrator  ExternalReset=either  InitialConditionSource=external  LimitOutput=on  UpperSaturationLimit=138  ShowStatePort=on
  Math Function : Math  Operator=pow  SaturateOnIntegerOverflow=on
  Subsystem : Subsystem
  Subsystem2 : Subsystem
  Sum : Sum  Inputs=|++
  Switch : Switch  Threshold=0.1
  v : Outport
  vnext : Outport  Port=2
  wires:
  win/1 -> Subsystem/5(win)
  vin/1 -> Subsystem/4(vin), Subsystem2/4(vin)
  Integrator/State -> vnext/1
  Constant1/1 -> Switch/3
  vno/1 -> Switch/1, Switch/2
  Sum/1 -> Subsystem/3(f(vno))
  Switch/1 -> Math Function/1
  Constant3/1 -> Sum/2
  Gain1/1 -> Sum/1
  Math Function/1 -> Gain1/1
  Constant2/1 -> Math Function/2
  I_st/1 -> Subsystem2/1(I_st)
  reset/1 -> Integrator/2
  vreset/1 -> IC/1
  Subsystem2/1(vint) -> Integrator/1
  Subsystem/1(vgain) -> Subsystem2/3(vgain)
  Integrator/1 -> Subsystem/2(v), v/1
  IC/1 -> Integrator/3
  q/1 -> Subsystem/1(q), Subsystem2/2(q)

== system heart_model/Heart Model/VENTRICLE/His_d (7)/Subsystem3 ==
  q : Inport
  vreset : Inport  Port=2
  reset : Inport  Port=3
  I_st : Inport  Port=4
  vno : Inport  Port=5
  vin : Inport  Port=6
  win : Inport  Port=7
  Constant1 : Constant  Value=0
  Constant2 : Constant  Value=1/6
  Constant3 : Constant
  Gain1 : Gain  Gain=13
  IC : InitialCondition  Value=0
  Integrator : Integrator  ExternalReset=either  InitialConditionSource=external  LimitOutput=on  UpperSaturationLimit=138  ShowStatePort=on
  Math Function : Math  Operator=pow  SaturateOnIntegerOverflow=on
  Subsystem : Subsystem
  Subsystem2 : Subsystem
  Sum : Sum  Inputs=|++
  Switch : Switch  Threshold=0.1
  v : Outport
  vnext : Outport  Port=2
  wires:
  win/1 -> Subsystem/5(win)
  vin/1 -> Subsystem/4(vin), Subsystem2/4(vin)
  Integrator/State -> vnext/1
  Constant1/1 -> Switch/3
  vno/1 -> Switch/1, Switch/2
  Sum/1 -> Subsystem/3(f(vno))
  Switch/1 -> Math Function/1
  Constant3/1 -> Sum/2
  Gain1/1 -> Sum/1
  Math Function/1 -> Gain1/1
  Constant2/1 -> Math Function/2
  I_st/1 -> Subsystem2/1(I_st)
  reset/1 -> Integrator/2
  vreset/1 -> IC/1
  Subsystem2/1(vint) -> Integrator/1
  Subsystem/1(vgain) -> Subsystem2/3(vgain)
  Integrator/1 -> Subsystem/2(v), v/1
  IC/1 -> Integrator/3
  q/1 -> Subsystem/1(q), Subsystem2/2(q)

== system heart_model/Heart Model/VENTRICLE/His_m (6)/Subsystem3 ==
  q : Inport
  vreset : Inport  Port=2
  reset : Inport  Port=3
  I_st : Inport  Port=4
  vno : Inport  Port=5
  vin : Inport  Port=6
  win : Inport  Port=7
  Constant1 : Constant  Value=0
  Constant2 : Constant  Value=1/6
  Constant3 : Constant
  Gain1 : Gain  Gain=13
  IC : InitialCondition  Value=0
  Integrator : Integrator  ExternalReset=either  InitialConditionSource=external  LimitOutput=on  UpperSaturationLimit=138  ShowStatePort=on
  Math Function : Math  Operator=pow  SaturateOnIntegerOverflow=on
  Subsystem : Subsystem
  Subsystem2 : Subsystem
  Sum : Sum  Inputs=|++
  Switch : Switch  Threshold=0.1
  v : Outport
  vnext : Outport  Port=2
  wires:
  win/1 -> Subsystem/5(win)
  vin/1 -> Subsystem/4(vin), Subsystem2/4(vin)
  Integrator/State -> vnext/1
  Constant1/1 -> Switch/3
  vno/1 -> Switch/1, Switch/2
  Sum/1 -> Subsystem/3(f(vno))
  Switch/1 -> Math Function/1
  Constant3/1 -> Sum/2
  Gain1/1 -> Sum/1
  Math Function/1 -> Gain1/1
  Constant2/1 -> Math Function/2
  I_st/1 -> Subsystem2/1(I_st)
  reset/1 -> Integrator/2
  vreset/1 -> IC/1
  Subsystem2/1(vint) -> Integrator/1
  Subsystem/1(vgain) -> Subsystem2/3(vgain)
  Integrator/1 -> Subsystem/2(v), v/1
  IC/1 -> Integrator/3
  q/1 -> Subsystem/1(q), Subsystem2/2(q)

== system heart_model/Heart Model/VENTRICLE/His_p (5)/Subsystem3 ==
  q : Inport
  vreset : Inport  Port=2
  reset : Inport  Port=3
  I_st : Inport  Port=4
  vno : Inport  Port=5
  vin : Inport  Port=6
  win : Inport  Port=7
  Constant1 : Constant  Value=0
  Constant2 : Constant  Value=1/6
  Constant3 : Constant
  Gain1 : Gain  Gain=13
  IC : InitialCondition  Value=0
  Integrator : Integrator  ExternalReset=either  InitialConditionSource=external  LimitOutput=on  UpperSaturationLimit=138  ShowStatePort=on
  Math Function : Math  Operator=pow  SaturateOnIntegerOverflow=on
  Subsystem : Subsystem
  Subsystem2 : Subsystem
  Sum : Sum  Inputs=|++
  Switch : Switch  Threshold=0.1
  v : Outport
  vnext : Outport  Port=2
  wires:
  win/1 -> Subsystem/5(win)
  vin/1 -> Subsystem/4(vin), Subsystem2/4(vin)
  Integrator/State -> vnext/1
  Constant1/1 -> Switch/3
  vno/1 -> Switch/1, Switch/2
  Sum/1 -> Subsystem/3(f(vno))
  Switch/1 -> Math Function/1
  Constant3/1 -> Sum/2
  Gain1/1 -> Sum/1
  Math Function/1 -> Gain1/1
  Constant2/1 -> Math Function/2
  I_st/1 -> Subsystem2/1(I_st)
  reset/1 -> Integrator/2
  vreset/1 -> IC/1
  Subsystem2/1(vint) -> Integrator/1
  Subsystem/1(vgain) -> Subsystem2/3(vgain)
  Integrator/1 -> Subsystem/2(v), v/1
  IC/1 -> Integrator/3
  q/1 -> Subsystem/1(q), Subsystem2/2(q)

== system heart_model/Heart Model/VENTRICLE/LBB (14)/Subsystem3 ==
  q : Inport
  vreset : Inport  Port=2
  reset : Inport  Port=3
  I_st : Inport  Port=4
  vno : Inport  Port=5
  vin : Inport  Port=6
  win : Inport  Port=7
  Constant1 : Constant  Value=0
  Constant2 : Constant  Value=1/6
  Constant3 : Constant
  Gain1 : Gain  Gain=13
  IC : InitialCondition  Value=0
  Integrator : Integrator  ExternalReset=either  InitialConditionSource=external  LimitOutput=on  UpperSaturationLimit=138  ShowStatePort=on
  Math Function : Math  Operator=pow  SaturateOnIntegerOverflow=on
  Subsystem : Subsystem
  Subsystem2 : Subsystem
  Sum : Sum  Inputs=|++
  Switch : Switch  Threshold=0.1
  v : Outport
  vnext : Outport  Port=2
  wires:
  win/1 -> Subsystem/5(win)
  vin/1 -> Subsystem/4(vin), Subsystem2/4(vin)
  Integrator/State -> vnext/1
  Constant1/1 -> Switch/3
  vno/1 -> Switch/1, Switch/2
  Sum/1 -> Subsystem/3(f(vno))
  Switch/1 -> Math Function/1
  Constant3/1 -> Sum/2
  Gain1/1 -> Sum/1
  Math Function/1 -> Gain1/1
  Constant2/1 -> Math Function/2
  I_st/1 -> Subsystem2/1(I_st)
  reset/1 -> Integrator/2
  vreset/1 -> IC/1
  Subsystem2/1(vint) -> Integrator/1
  Subsystem/1(vgain) -> Subsystem2/3(vgain)
  Integrator/1 -> Subsystem/2(v), v/1
  IC/1 -> Integrator/3
  q/1 -> Subsystem/1(q), Subsystem2/2(q)

== system heart_model/Heart Model/VENTRICLE/LBB_m (13)/Subsystem3 ==
  q : Inport
  vreset : Inport  Port=2
  reset : Inport  Port=3
  I_st : Inport  Port=4
  vno : Inport  Port=5
  vin : Inport  Port=6
  win : Inport  Port=7
  Constant1 : Constant  Value=0
  Constant2 : Constant  Value=1/6
  Constant3 : Constant
  Gain1 : Gain  Gain=13
  IC : InitialCondition  Value=0
  Integrator : Integrator  ExternalReset=either  InitialConditionSource=external  LimitOutput=on  UpperSaturationLimit=138  ShowStatePort=on
  Math Function : Math  Operator=pow  SaturateOnIntegerOverflow=on
  Subsystem : Subsystem
  Subsystem2 : Subsystem
  Sum : Sum  Inputs=|++
  Switch : Switch  Threshold=0.1
  v : Outport
  vnext : Outport  Port=2
  wires:
  win/1 -> Subsystem/5(win)
  vin/1 -> Subsystem/4(vin), Subsystem2/4(vin)
  Integrator/State -> vnext/1
  Constant1/1 -> Switch/3
  vno/1 -> Switch/1, Switch/2
  Sum/1 -> Subsystem/3(f(vno))
  Switch/1 -> Math Function/1
  Constant3/1 -> Sum/2
  Gain1/1 -> Sum/1
  Math Function/1 -> Gain1/1
  Constant2/1 -> Math Function/2
  I_st/1 -> Subsystem2/1(I_st)
  reset/1 -> Integrator/2
  vreset/1 -> IC/1
  Subsystem2/1(vint) -> Integrator/1
  Subsystem/1(vgain) -> Subsystem2/3(vgain)
  Integrator/1 -> Subsystem/2(v), v/1
  IC/1 -> Integrator/3
  q/1 -> Subsystem/1(q), Subsystem2/2(q)

== system heart_model/Heart Model/VENTRICLE/LV (20)/Subsystem3 ==
  q : Inport
  vreset : Inport  Port=2
  reset : Inport  Port=3
  I_st : Inport  Port=4
  vno : Inport  Port=5
  vin : Inport  Port=6
  win : Inport  Port=7
  Constant1 : Constant  Value=0
  Constant2 : Constant  Value=1/6
  Constant3 : Constant
  Gain1 : Gain  Gain=13
  IC : InitialCondition  Value=0
  Integrator : Integrator  ExternalReset=either  InitialConditionSource=external  LimitOutput=on  UpperSaturationLimit=138  ShowStatePort=on
  Math Function : Math  Operator=pow  SaturateOnIntegerOverflow=on
  Subsystem : Subsystem
  Subsystem2 : Subsystem
  Sum : Sum  Inputs=|++
  Switch : Switch  Threshold=0.1
  v : Outport
  vnext : Outport  Port=2
  wires:
  win/1 -> Subsystem/5(win)
  vin/1 -> Subsystem/4(vin), Subsystem2/4(vin)
  Integrator/State -> vnext/1
  Constant1/1 -> Switch/3
  vno/1 -> Switch/1, Switch/2
  Sum/1 -> Subsystem/3(f(vno))
  Switch/1 -> Math Function/1
  Constant3/1 -> Sum/2
  Gain1/1 -> Sum/1
  Math Function/1 -> Gain1/1
  Constant2/1 -> Math Function/2
  I_st/1 -> Subsystem2/1(I_st)
  reset/1 -> Integrator/2
  vreset/1 -> IC/1
  Subsystem2/1(vint) -> Integrator/1
  Subsystem/1(vgain) -> Subsystem2/3(vgain)
  Integrator/1 -> Subsystem/2(v), v/1
  IC/1 -> Integrator/3
  q/1 -> Subsystem/1(q), Subsystem2/2(q)

== system heart_model/Heart Model/VENTRICLE/LVA (16)/Subsystem3 ==
  q : Inport
  vreset : Inport  Port=2
  reset : Inport  Port=3
  I_st : Inport  Port=4
  vno : Inport  Port=5
  vin : Inport  Port=6
  win : Inport  Port=7
  Constant1 : Constant  Value=0
  Constant2 : Constant  Value=1/6
  Constant3 : Constant
  Gain1 : Gain  Gain=13
  IC : InitialCondition  Value=0
  Integrator : Integrator  ExternalReset=either  InitialConditionSource=external  LimitOutput=on  UpperSaturationLimit=138  ShowStatePort=on
  Math Function : Math  Operator=pow  SaturateOnIntegerOverflow=on
  Subsystem : Subsystem
  Subsystem2 : Subsystem
  Sum : Sum  Inputs=|++
  Switch : Switch  Threshold=0.1
  v : Outport
  vnext : Outport  Port=2
  wires:
  win/1 -> Subsystem/5(win)
  vin/1 -> Subsystem/4(vin), Subsystem2/4(vin)
  Integrator/State -> vnext/1
  Constant1/1 -> Switch/3
  vno/1 -> Switch/1, Switch/2
  Sum/1 -> Subsystem/3(f(vno))
  Switch/1 -> Math Function/1
  Constant3/1 -> Sum/2
  Gain1/1 -> Sum/1
  Math Function/1 -> Gain1/1
  Constant2/1 -> Math Function/2
  I_st/1 -> Subsystem2/1(I_st)
  reset/1 -> Integrator/2
  vreset/1 -> IC/1
  Subsystem2/1(vint) -> Integrator/1
  Subsystem/1(vgain) -> Subsystem2/3(vgain)
  Integrator/1 -> Subsystem/2(v), v/1
  IC/1 -> Integrator/3
  q/1 -> Subsystem/1(q), Subsystem2/2(q)

== system heart_model/Heart Model/VENTRICLE/LV_m (19)/Subsystem3 ==
  q : Inport
  vreset : Inport  Port=2
  reset : Inport  Port=3
  I_st : Inport  Port=4
  vno : Inport  Port=5
  vin : Inport  Port=6
  win : Inport  Port=7
  Constant1 : Constant  Value=0
  Constant2 : Constant  Value=1/6
  Constant3 : Constant
  Gain1 : Gain  Gain=13
  IC : InitialCondition  Value=0
  Integrator : Integrator  ExternalReset=either  InitialConditionSource=external  LimitOutput=on  UpperSaturationLimit=138  ShowStatePort=on
  Math Function : Math  Operator=pow  SaturateOnIntegerOverflow=on
  Subsystem : Subsystem
  Subsystem2 : Subsystem
  Sum : Sum  Inputs=|++
  Switch : Switch  Threshold=0.1
  v : Outport
  vnext : Outport  Port=2
  wires:
  win/1 -> Subsystem/5(win)
  vin/1 -> Subsystem/4(vin), Subsystem2/4(vin)
  Integrator/State -> vnext/1
  Constant1/1 -> Switch/3
  vno/1 -> Switch/1, Switch/2
  Sum/1 -> Subsystem/3(f(vno))
  Switch/1 -> Math Function/1
  Constant3/1 -> Sum/2
  Gain1/1 -> Sum/1
  Math Function/1 -> Gain1/1
  Constant2/1 -> Math Function/2
  I_st/1 -> Subsystem2/1(I_st)
  reset/1 -> Integrator/2
  vreset/1 -> IC/1
  Subsystem2/1(vint) -> Integrator/1
  Subsystem/1(vgain) -> Subsystem2/3(vgain)
  Integrator/1 -> Subsystem/2(v), v/1
  IC/1 -> Integrator/3
  q/1 -> Subsystem/1(q), Subsystem2/2(q)

== system heart_model/Heart Model/VENTRICLE/RBB (12)/Subsystem3 ==
  q : Inport
  vreset : Inport  Port=2
  reset : Inport  Port=3
  I_st : Inport  Port=4
  vno : Inport  Port=5
  vin : Inport  Port=6
  win : Inport  Port=7
  Constant1 : Constant  Value=0
  Constant2 : Constant  Value=1/6
  Constant3 : Constant
  Gain1 : Gain  Gain=13
  IC : InitialCondition  Value=0
  Integrator : Integrator  ExternalReset=either  InitialConditionSource=external  LimitOutput=on  UpperSaturationLimit=138  ShowStatePort=on
  Math Function : Math  Operator=pow  SaturateOnIntegerOverflow=on
  Subsystem : Subsystem
  Subsystem2 : Subsystem
  Sum : Sum  Inputs=|++
  Switch : Switch  Threshold=0.1
  v : Outport
  vnext : Outport  Port=2
  wires:
  win/1 -> Subsystem/5(win)
  vin/1 -> Subsystem/4(vin), Subsystem2/4(vin)
  Integrator/State -> vnext/1
  Constant1/1 -> Switch/3
  vno/1 -> Switch/1, Switch/2
  Sum/1 -> Subsystem/3(f(vno))
  Switch/1 -> Math Function/1
  Constant3/1 -> Sum/2
  Gain1/1 -> Sum/1
  Math Function/1 -> Gain1/1
  Constant2/1 -> Math Function/2
  I_st/1 -> Subsystem2/1(I_st)
  reset/1 -> Integrator/2
  vreset/1 -> IC/1
  Subsystem2/1(vint) -> Integrator/1
  Subsystem/1(vgain) -> Subsystem2/3(vgain)
  Integrator/1 -> Subsystem/2(v), v/1
  IC/1 -> Integrator/3
  q/1 -> Subsystem/1(q), Subsystem2/2(q)
